simulink model "untitled"  (R2016a)
settings: Solver=VariableStepAuto  StartTime=0.0  StopTime=1000.0  RelTol=1e-3
settings Model: Creator=Ivan Varabei  LastModifiedBy=Ivan Varabei

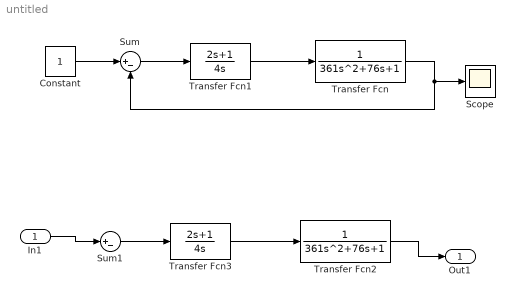
== system untitled ==
  In1 : Inport
  Constant : Constant
  Scope : Scope
  Sum : Sum  Inputs=|+-
  Sum1 : Sum  Inputs=|+-
  Transfer Fcn : TransferFcn  Denominator=[361 76 1]
  Transfer Fcn1 : TransferFcn  Numerator=[2 1]  Denominator=[4 0]
  Transfer Fcn2 : TransferFcn  Denominator=[361 76 1]
  Transfer Fcn3 : TransferFcn  Numerator=[2 1]  Denominator=[4 0]
  Out1 : Outport
  wires:
  Transfer Fcn/1 -> Sum/2, Scope/1
  Transfer Fcn1/1 -> Transfer Fcn/1
  Sum/1 -> Transfer Fcn1/1
  Constant/1 -> Sum/1
  Transfer Fcn3/1 -> Transfer Fcn2/1
  Sum1/1 -> Transfer Fcn3/1
  Transfer Fcn2/1 -> Out1/1
  In1/1 -> Sum1/1
